simulink library "BLDC_controller_Lib"  (R2017b)
settings: Solver=VariableStepAuto  StartTime=0.0  StopTime=10.0  RelTol=1e-3
undefined symbols (not defined in the file): a_elecAngle, a_elecPeriod, a_phaAdv_M1, b_phaAdvEna, cf_speedCoef, cf_speedFilt, CTRL_COMM, dz_counterHi, dz_counterLo, n_commAcvLo, n_commDeacvHi, n_motPhaAdvEna, r_commDCDeacv, r_sin3PhaA_M1, r_sin3PhaB_M1, r_sin3PhaC_M1, r_sinPhaA_M1, r_sinPhaB_M1, r_sinPhaC_M1, r_trapPhaA_M1, r_trapPhaB_M1, r_trapPhaC_M1, vec_hallToPos, z_commutMap_M1, z_ctrlTypSel, z_maxCntRst
libraries: BLDC_controller_Lib x2, simulink x1
settings Model: Creator=37ef  LastModifiedBy=eferu

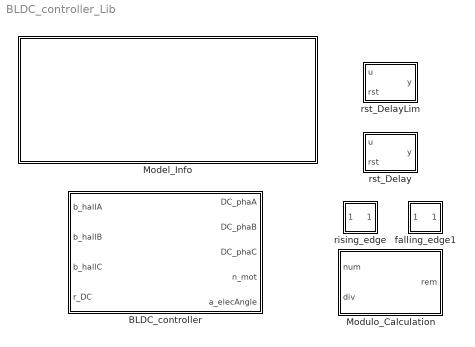
== system BLDC_controller_Lib ==
  BLDC_controller : Subsystem  SystemSampleTime=1e-5
  Model_Info : Subsystem
      mask DialogControl DescGroupVar Prompt: Model info
      mask DialogControl DescTextVar Prompt: This mask gives quick information about the model.
      mask Display:
      | info = Simulink.MDLInfo(bdroot);
      | file = dir([bdroot '.slx']);
      | % image('logo.png', [0.48, 0.55, 0.5, 0.4]);
      | text(0.05, 0.5, [...
      |         'MODEL INFO \n\n' ...
      |         'Version: ' info.ModelVersion '\n' ...
      |         'Author: ' 'Emanuel Feru' '\n' ...
      |         'Last modified by: ' info.LastModifiedBy '\n' ...
      |         'Last update: ' file.date '\n\n'], ...
      |         'horizontalAlignment', 'left', ...
      |         'verticalAlignment', 'middle');
      | 
      | color('blue');
      | text(0.95, 0.08, [...
      |         'Copyright © 2019 Emanuel FERU'], ...
      |         'horizontalAlignment', 'right', ...
      |         'verticalAlignment', 'bottom');
  Modulo_Calculation : Subsystem
  falling_edge1 : Subsystem  StopFcn=%tagged  TreatAsAtomicUnit=on  mask(Falling edge detection){}
      mask help:
      | Falling edge detection for a logic signal.
      | When a falling edge on the input signal is detected, the output switches to 1 during one time step.
      settings: RTWSystemCode=Nonreusable function
      mask Display: plot(0,0,100,100, [20 50 50 80], [90 90 10 10], [40 50 60], [55 45 55] )
  rising_edge : Subsystem  StopFcn=%tagged  TreatAsAtomicUnit=on  mask(Rising edge detection){}
      mask help:
      | Rising edge detection for a logic signal.
      | When a rising edge on the input signal is detected, the output switches to 1 during one time step.
      settings: RTWSystemCode=Nonreusable function
      mask Display: plot(0,0,100,100, [20 50 50 80], [10 10 90 90], [40 50 60], [45 55 45] )
  rst_Delay : Subsystem
      mask Display: dpoly(1,[1 0],'z')
  rst_DelayLim : Subsystem  mask{z_cntMaxLim=200}
      mask prompts: z_cntMaxLim "Maximum counter limit"
      mask Display: dpoly(1,[1 0],'z')

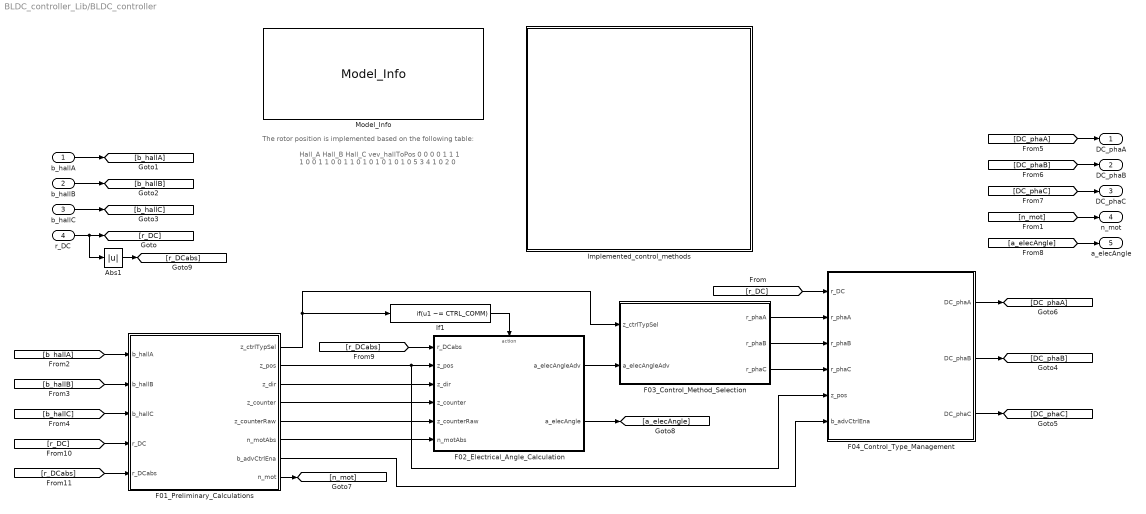
== system BLDC_controller_Lib/BLDC_controller ==
  note: Hall_A
      | Hall_B
      | Hall_C
      | vev_hallToPos
      |
      | 0
      | 0
      | 0
      | 0
      | 1
      | 1
      | 1
      | 1
      | 0
      | 0
      | 1
      | 1
      | 0
      | 0
      | 1
      | 1
      | 0
      | 1
      | 0
      | 1
      | 0
      | 1
      | 0
      | 1
      | 0
      | 5
      | 3
      | 4
      | 1
      | 0
      | 2
      | 0
  note: The rotor position is implemented based on the following table:
  "b_hallA " : Inport
  b_hallB : Inport  Port=2
  b_hallC : Inport  Port=3
  r_DC : Inport  Port=4
  Abs1 : Abs  OutDataTypeStr=Inherit: Inherit via back propagation  RndMeth=Zero
  F01_Preliminary_Calculations : Subsystem
  F02_Electrical_Angle_Calculation : Subsystem
  F03_Control_Method_Selection : Subsystem
  F04_Control_Type_Management : Subsystem
  If1 : If  IfExpression=u1 ~= CTRL_COMM  ShowElse=off
  Implemented_control_methods : Subsystem
      mask Display: image('control_methods.png')
  Model_Info : BLDC_controller_Lib/Model_Info
  DC_phaA : Outport
  DC_phaB : Outport  Port=2
  DC_phaC : Outport  Port=3
  n_mot : Outport  Port=4
  a_elecAngle : Outport  Port=5
  wires:
  F01_Preliminary_Calculations/6(n_motAbs) -> F02_Electrical_Angle_Calculation/6(n_motAbs)
  [r_DCabs] -> F01_Preliminary_Calculations/5(r_DCabs)
  Abs1/1 -> [r_DCabs]
  F01_Preliminary_Calculations/5(z_counterRaw) -> F02_Electrical_Angle_Calculation/5(z_counterRaw)
  F01_Preliminary_Calculations/4(z_counter) -> F02_Electrical_Angle_Calculation/4(z_counter)
  F01_Preliminary_Calculations/7(b_advCtrlEna) -> F04_Control_Type_Management/6(b_advCtrlEna)
  [r_DC] -> F01_Preliminary_Calculations/4(r_DC)
  [r_DCabs] -> F02_Electrical_Angle_Calculation/1(r_DCabs)
  F02_Electrical_Angle_Calculation/2(a_elecAngle) -> [a_elecAngle]
  [a_elecAngle] -> a_elecAngle/1
  r_DC/1 -> Abs1/1, [r_DC]
  [DC_phaC] -> DC_phaC/1
  [DC_phaB] -> DC_phaB/1
  F04_Control_Type_Management/3("DC_phaC ") -> [DC_phaC]
  F04_Control_Type_Management/2(DC_phaB) -> [DC_phaB]
  F04_Control_Type_Management/1(DC_phaA) -> [DC_phaA]
  [r_DC] -> F04_Control_Type_Management/1(r_DC)
  F03_Control_Method_Selection/3("r_phaC ") -> F04_Control_Type_Management/4(r_phaC)
  F03_Control_Method_Selection/2(r_phaB) -> F04_Control_Type_Management/3(r_phaB)
  F03_Control_Method_Selection/1(r_phaA) -> F04_Control_Type_Management/2(r_phaA)
  F02_Electrical_Angle_Calculation/1(a_elecAngleAdv) -> F03_Control_Method_Selection/2(a_elecAngleAdv)
  If1/1 -> F02_Electrical_Angle_Calculation/Action
  F01_Preliminary_Calculations/1(z_ctrlTypSel) -> If1/1, F03_Control_Method_Selection/1(z_ctrlTypSel)
  F01_Preliminary_Calculations/8("n_mot ") -> [n_mot]
  F01_Preliminary_Calculations/3(z_dir) -> F02_Electrical_Angle_Calculation/3(z_dir)
  F01_Preliminary_Calculations/2(z_pos) -> F02_Electrical_Angle_Calculation/2(z_pos), F04_Control_Type_Management/5(z_pos)
  [b_hallB] -> F01_Preliminary_Calculations/2(b_hallB)
  [b_hallC] -> F01_Preliminary_Calculations/3(b_hallC)
  [b_hallA] -> F01_Preliminary_Calculations/1(b_hallA)
  [DC_phaA] -> DC_phaA/1
  [n_mot] -> n_mot/1
  b_hallC/1 -> [b_hallC]
  b_hallB/1 -> [b_hallB]
  "b_hallA "/1 -> [b_hallA]

== system BLDC_controller_Lib/Model_Info ==

== system BLDC_controller_Lib/Modulo_Calculation ==
  note: Modulo implementation: rem = num - div*(num/div)
      | Note : Division and multiplier has the setting 'Floor'
  num : Inport
  div : Inport  Port=2
  Divide2 : Product  Inputs=*/  OutDataTypeStr=Inherit: Same as first input
  Divide3 : Product  Inputs=**  OutDataTypeStr=Inherit: Same as first input
  Sum3 : Sum  Inputs=|+-  RndMeth=Simplest  OutDataTypeStr=Inherit: Same as first input
  rem : Outport
  wires:
  num/1 -> Sum3/1, Divide2/1
  Sum3/1 -> rem/1
  Divide3/1 -> Sum3/2
  div/1 -> Divide3/2, Divide2/2
  Divide2/1 -> Divide3/1

== system BLDC_controller_Lib/falling_edge1 ==
  Signal : Inport
  Logical Operator : Logic  Tag=struct('inputs','2','comment',struct('text','','placement',1),'logdata',struct('maxnumvals',inf,'plotchannels',[],'loggingmode',3,'channels',1),'operator','AND','output',struct('variable','','description','','name','$S_$B','address','','class','default','type','Bool','unit',''),'scalingvalid',0,'date',733067.68453166669)  OutDataTypeStr=boolean
  Logical Operator1 : Logic  Tag=struct('inputs','1','comment',struct('text','','placement',1),'logdata',struct('maxnumvals',inf,'plotchannels',[],'loggingmode',3,'channels',1),'operator','NOT','output',struct('variable','','description','','name','$S_$B','address','','class','default','type','Bool','unit',''),'scalingvalid',0,'date',733067.68453201384)  Operator=NOT  Inputs=1  OutDataTypeStr=boolean
  UnitDelay : UnitDelay  SampleTime=-1
      settings: AttributesFormatString=Te = %<SampleTime>\nIni=%<X0>
  Out : Outport
  wires:
  UnitDelay/1 -> Logical Operator/2
  Logical Operator1/1 -> Logical Operator/1
  Signal/1 -> UnitDelay/1, Logical Operator1/1
  Logical Operator/1 -> Out/1

== system BLDC_controller_Lib/rising_edge ==
  Signal : Inport
  Logical Operator : Logic  Tag=struct('inputs','2','comment',struct('text','','placement',1),'logdata',struct('maxnumvals',inf,'plotchannels',[],'loggingmode',3,'channels',1),'operator','AND','output',struct('variable','','description','','name','$S_$B','address','','class','default','type','Bool','unit',''),'scalingvalid',0,'date',733067.68458487268)  OutDataTypeStr=boolean
  Logical Operator1 : Logic  Tag=struct('inputs','1','comment',struct('text','','placement',1),'logdata',struct('maxnumvals',inf,'plotchannels',[],'loggingmode',3,'channels',1),'operator','NOT','output',struct('variable','','description','','name','$S_$B','address','','class','default','type','Bool','unit',''),'scalingvalid',0,'date',733067.68458533566)  Operator=NOT  Inputs=1  OutDataTypeStr=boolean
  UnitDelay : UnitDelay  SampleTime=-1
      settings: AttributesFormatString=Te = %<SampleTime>\nIni=%<X0>
  Out : Outport
  wires:
  UnitDelay/1 -> Logical Operator1/1
  Logical Operator1/1 -> Logical Operator/2
  Signal/1 -> Logical Operator/1, UnitDelay/1
  Logical Operator/1 -> Out/1

== system BLDC_controller_Lib/rst_Delay ==
  u : Inport
  rst : Inport  Port=2
  Constant23 : Constant  Value=0  OutDataTypeStr=Inherit: Inherit via back propagation
  Switch1 : Switch  Criteria=u2 ~= 0  OutDataTypeStr=Inherit: Inherit via back propagation  RndMeth=Simplest
  UnitDelay1 : UnitDelay  SampleTime=-1
  y : Outport
  wires:
  Switch1/1 -> y/1
  u/1 -> UnitDelay1/1
  UnitDelay1/1 -> Switch1/3
  rst/1 -> Switch1/2
  Constant23/1 -> Switch1/1

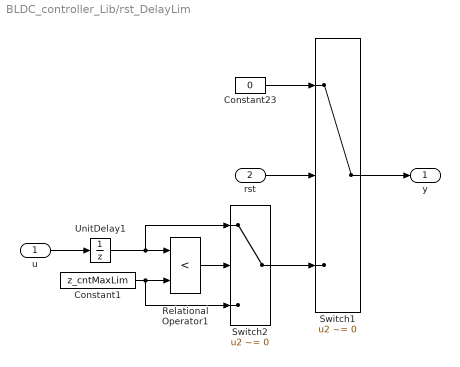
== system BLDC_controller_Lib/rst_DelayLim ==
  u : Inport
  rst : Inport  Port=2
  Constant1 : Constant  Value=z_cntMaxLim  OutDataTypeStr=Inherit: Inherit via back propagation
  Constant23 : Constant  Value=0  OutDataTypeStr=Inherit: Inherit via back propagation
  Relational Operator1 : RelationalOperator  Operator=<  OutDataTypeStr=boolean  RndMeth=Simplest
  Switch1 : Switch  Criteria=u2 ~= 0  OutDataTypeStr=Inherit: Inherit via back propagation  RndMeth=Simplest
  Switch2 : Switch  Criteria=u2 ~= 0  OutDataTypeStr=Inherit: Inherit via back propagation  RndMeth=Simplest
  UnitDelay1 : UnitDelay  InitialCondition=z_cntMaxLim  SampleTime=-1
  y : Outport
  wires:
  Switch1/1 -> y/1
  u/1 -> UnitDelay1/1
  rst/1 -> Switch1/2
  Constant23/1 -> Switch1/1
  UnitDelay1/1 -> Switch2/1, Relational Operator1/1
  Constant1/1 -> Switch2/3, Relational Operator1/2
  Relational Operator1/1 -> Switch2/2
  Switch2/1 -> Switch1/3

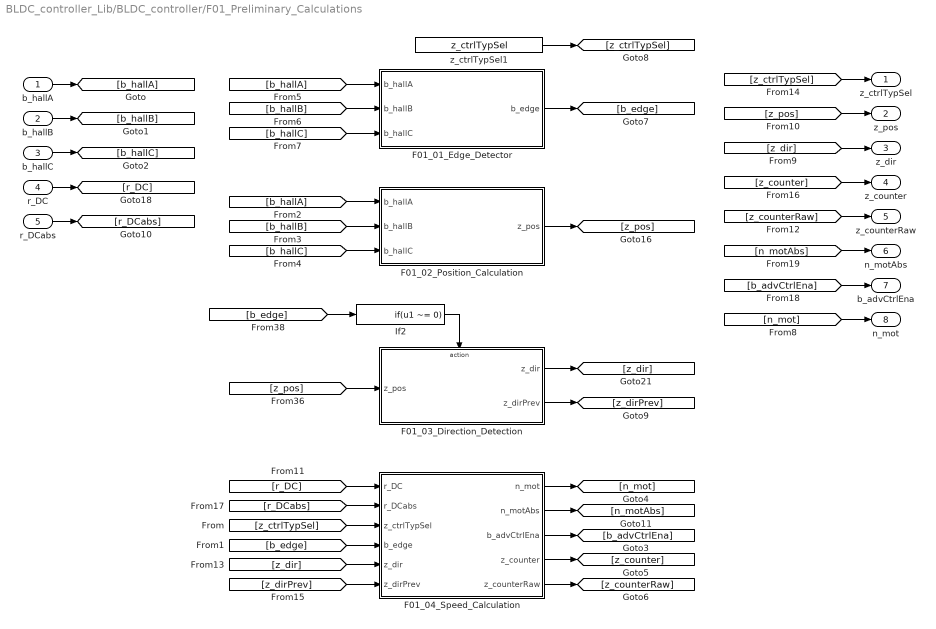
== system BLDC_controller_Lib/BLDC_controller/F01_Preliminary_Calculations ==
  b_hallA : Inport
  b_hallB : Inport  Port=2
  b_hallC : Inport  Port=3
  r_DC : Inport  Port=4
  r_DCabs : Inport  Port=5
  F01_01_Edge_Detector : Subsystem
  F01_02_Position_Calculation : Subsystem
  F01_03_Direction_Detection : Subsystem
  F01_04_Speed_Calculation : Subsystem
  If2 : If  IfExpression=u1 ~= 0  ShowElse=off
  z_ctrlTypSel1 : Constant  Value=z_ctrlTypSel  OutDataTypeStr=uint8
  z_ctrlTypSel : Outport  OutputWhenDisabled=reset  InitialOutput=0
  z_pos : Outport  Port=2  OutputWhenDisabled=reset  InitialOutput=0
  z_dir : Outport  Port=3  OutputWhenDisabled=reset  InitialOutput=0
  z_counter : Outport  Port=4  OutputWhenDisabled=reset  InitialOutput=0
  z_counterRaw : Outport  Port=5  OutputWhenDisabled=reset  InitialOutput=0
  n_motAbs : Outport  Port=6  OutputWhenDisabled=reset  InitialOutput=0
  b_advCtrlEna : Outport  Port=7
  "n_mot " : Outport  Port=8  OutputWhenDisabled=reset  InitialOutput=0
  wires:
  [n_motAbs] -> n_motAbs/1
  F01_04_Speed_Calculation/2(n_motAbs) -> [n_motAbs]
  [r_DCabs] -> F01_04_Speed_Calculation/2(r_DCabs)
  r_DCabs/1 -> [r_DCabs]
  [z_dirPrev] -> F01_04_Speed_Calculation/6(z_dirPrev)
  F01_03_Direction_Detection/2(z_dirPrev) -> [z_dirPrev]
  F01_04_Speed_Calculation/5(z_counterRaw) -> [z_counterRaw]
  F01_04_Speed_Calculation/4(z_counter) -> [z_counter]
  [z_counterRaw] -> z_counterRaw/1
  [z_counter] -> z_counter/1
  F01_04_Speed_Calculation/3(b_advCtrlEna) -> [b_advCtrlEna]
  [b_advCtrlEna] -> b_advCtrlEna/1
  [r_DC] -> F01_04_Speed_Calculation/1(r_DC)
  [z_ctrlTypSel] -> F01_04_Speed_Calculation/3(z_ctrlTypSel)
  r_DC/1 -> [r_DC]
  z_ctrlTypSel1/1 -> [z_ctrlTypSel]
  [z_ctrlTypSel] -> z_ctrlTypSel/1
  [z_dir] -> F01_04_Speed_Calculation/5(z_dir)
  [z_pos] -> z_pos/1
  [z_dir] -> z_dir/1
  [n_mot] -> "n_mot "/1
  F01_04_Speed_Calculation/1(n_mot) -> [n_mot]
  [b_edge] -> F01_04_Speed_Calculation/4(b_edge)
  F01_02_Position_Calculation/1("z_pos ") -> [z_pos]
  [b_hallA] -> F01_02_Position_Calculation/1(b_hallA)
  [b_hallB] -> F01_02_Position_Calculation/2(b_hallB)
  [b_hallC] -> F01_02_Position_Calculation/3(b_hallC)
  b_hallC/1 -> [b_hallC]
  b_hallB/1 -> [b_hallB]
  b_hallA/1 -> [b_hallA]
  [b_hallC] -> F01_01_Edge_Detector/3(b_hallC)
  [b_hallB] -> F01_01_Edge_Detector/2(b_hallB)
  F01_03_Direction_Detection/1(z_dir) -> [z_dir]
  F01_01_Edge_Detector/1("b_edge ") -> [b_edge]
  [b_hallA] -> F01_01_Edge_Detector/1(b_hallA)
  [z_pos] -> F01_03_Direction_Detection/1(z_pos)
  [b_edge] -> If2/1
  If2/1 -> F01_03_Direction_Detection/Action

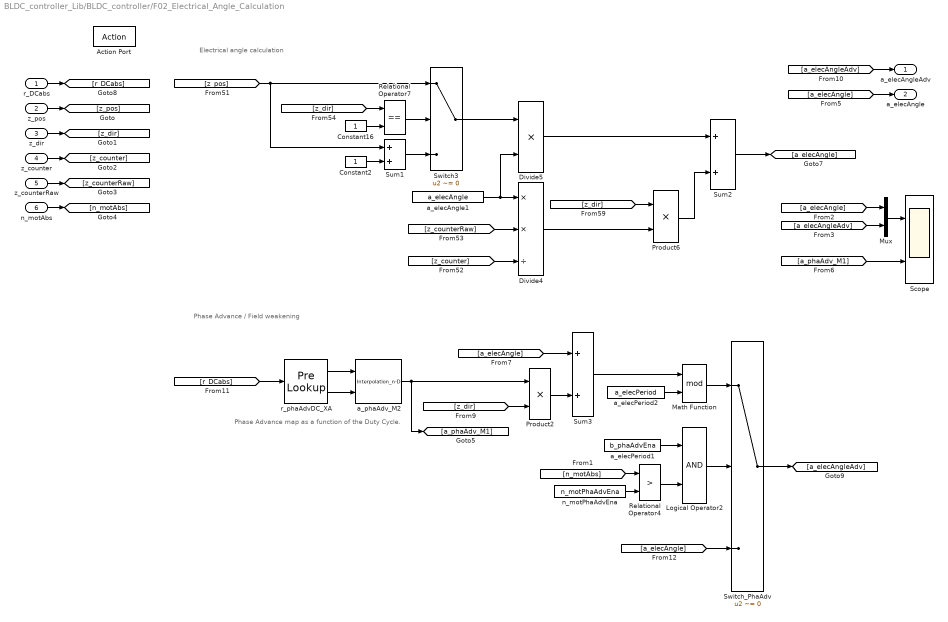
== system BLDC_controller_Lib/BLDC_controller/F02_Electrical_Angle_Calculation ==
  note: Phase Advance map as a function of the Duty Cycle.
  note: Phase Advance / Field weakening
  note: Electrical angle calculation
  r_DCabs : Inport
  z_pos : Inport  Port=2
  z_dir : Inport  Port=3
  z_counter : Inport  Port=4
  z_counterRaw : Inport  Port=5
  n_motAbs : Inport  Port=6
  Action Port : ActionPort
  Constant16 : Constant  OutDataTypeStr=Inherit: Inherit via back propagation
  Constant2 : Constant  OutDataTypeStr=Inherit: Inherit via back propagation
  Divide4 : Product  Inputs=**/  OutDataTypeStr=int32  RndMeth=Simplest
  Divide5 : Product  Inputs=**  OutDataTypeStr=int32  RndMeth=Simplest
  Logical Operator2 : Logic  AllPortsSameDT=off  OutDataTypeStr=boolean
  Math Function : Math  Operator=mod  SaturateOnIntegerOverflow=on
  Mux : Mux  Inputs=2
  Product2 : Product  RndMeth=Simplest  OutDataTypeStr=Inherit: Same as first input
  Product6 : Product  OutDataTypeStr=Inherit: Inherit via back propagation  RndMeth=Simplest
  Relational Operator4 : RelationalOperator  Operator=>  OutDataTypeStr=boolean  RndMeth=Simplest
  Relational Operator7 : RelationalOperator  Operator===  OutDataTypeStr=boolean  RndMeth=Simplest
  Scope : Scope  NumInputPorts=2
  Sum1 : Sum  RndMeth=Simplest  OutDataTypeStr=Inherit: Same as first input
  Sum2 : Sum  RndMeth=Simplest  OutDataTypeStr=Inherit: Same as first input
  Sum3 : Sum  RndMeth=Simplest  OutDataTypeStr=Inherit: Same as first input
  Switch3 : Switch  Criteria=u2 ~= 0  OutDataTypeStr=Inherit: Inherit via back propagation  RndMeth=Zero
  Switch_PhaAdv : Switch  Criteria=u2 ~= 0  OutDataTypeStr=Inherit: Inherit via back propagation  RndMeth=Zero
  a_elecAngle1 : Constant  Value=a_elecAngle  OutDataTypeStr=int32
  a_elecPeriod1 : Constant  Value=b_phaAdvEna  OutDataTypeStr=boolean
  a_elecPeriod2 : Constant  Value=a_elecPeriod  OutDataTypeStr=Inherit: Inherit via back propagation
  a_phaAdv_M2 : Interpolation_n-D  NumberOfTableDimensions=1  Table=a_phaAdv_M1  ExtrapMethod=Clip  OutDataTypeStr=int16  InternalRulePriority=Speed  RndMeth=Simplest
      settings: InputPortMap=u0,u1
  n_motPhaAdvEna : Constant  Value=n_motPhaAdvEna  OutDataTypeStr=Inherit: Inherit via back propagation
  r_phaAdvDC_XA : PreLookup  BreakpointsData=r_phaAdvDC_XA  IndexSearchMethod=Evenly spaced points  BeginIndexSearchUsingPreviousIndexResult=on  IndexDataTypeStr=uint8  RndMeth=Simplest
  a_elecAngleAdv : Outport  OutputWhenDisabled=reset  InitialOutput=0
  a_elecAngle : Outport  Port=2  OutputWhenDisabled=reset  InitialOutput=0
  wires:
  n_motAbs/1 -> [n_motAbs]
  Logical Operator2/1 -> Switch_PhaAdv/2
  Relational Operator4/1 -> Logical Operator2/2
  [n_motAbs] -> Relational Operator4/1
  n_motPhaAdvEna/1 -> Relational Operator4/2
  a_elecPeriod1/1 -> Logical Operator2/1
  Divide5/1 -> Sum2/1
  Divide4/1 -> Product6/2
  Sum1/1 -> Switch3/3
  [z_dir] -> Relational Operator7/1
  a_elecAngle1/1 -> Divide4/1, Divide5/2
  Constant16/1 -> Relational Operator7/2
  Relational Operator7/1 -> Switch3/2
  Product6/1 -> Sum2/2
  [z_counter] -> Divide4/3
  Constant2/1 -> Sum1/2
  [z_pos] -> Sum1/1, Switch3/1
  Sum2/1 -> [a_elecAngle]
  [z_dir] -> Product6/1
  Switch3/1 -> Divide5/1
  [z_counterRaw] -> Divide4/2
  z_counter/1 -> [z_counter]
  z_counterRaw/1 -> [z_counterRaw]
  Sum3/1 -> Math Function/1
  Math Function/1 -> Switch_PhaAdv/1
  a_elecPeriod2/1 -> Math Function/2
  [r_DCabs] -> r_phaAdvDC_XA/1
  [a_elecAngle] -> Sum3/1
  Product2/1 -> Sum3/2
  Switch_PhaAdv/1 -> [a_elecAngleAdv]
  r_DCabs/1 -> [r_DCabs]
  [a_elecAngle] -> Switch_PhaAdv/3
  r_phaAdvDC_XA/1 -> a_phaAdv_M2/1
  r_phaAdvDC_XA/2 -> a_phaAdv_M2/2
  [a_phaAdv_M1] -> Scope/2
  [a_elecAngleAdv] -> a_elecAngleAdv/1
  [a_elecAngle] -> a_elecAngle/1
  [a_elecAngleAdv] -> Mux/2
  [a_elecAngle] -> Mux/1
  Mux/1 -> Scope/1
  z_dir/1 -> [z_dir]
  z_pos/1 -> [z_pos]
  [z_dir] -> Product2/2
  a_phaAdv_M2/1 -> Product2/1, [a_phaAdv_M1]

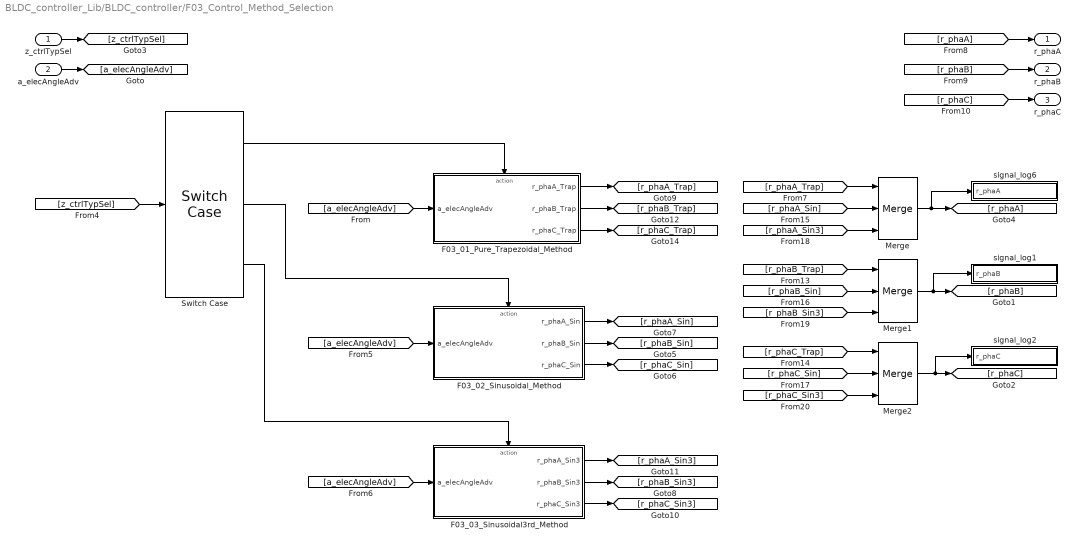
== system BLDC_controller_Lib/BLDC_controller/F03_Control_Method_Selection ==
  z_ctrlTypSel : Inport
  a_elecAngleAdv : Inport  Port=2
  F03_01_Pure_Trapezoidal_Method : Subsystem
  F03_02_Sinusoidal_Method : Subsystem
  F03_03_Sinusoidal3rd_Method : Subsystem
  Merge : Merge  Inputs=3
  Merge1 : Merge  Inputs=3
  Merge2 : Merge  Inputs=3
  Switch Case : SwitchCase  CaseConditions={CTRL_TRAP, CTRL_SIN, CTRL_SIN3}  ShowDefaultCase=off
  signal_log1 : Subsystem
  signal_log2 : Subsystem
  signal_log6 : Subsystem
  r_phaA : Outport  OutputWhenDisabled=reset  InitialOutput=0
  r_phaB : Outport  Port=2  OutputWhenDisabled=reset  InitialOutput=0
  "r_phaC " : Outport  Port=3  OutputWhenDisabled=reset  InitialOutput=0
  wires:
  [r_phaC_Sin3] -> Merge2/3
  [r_phaC_Sin] -> Merge2/2
  [r_phaB_Sin3] -> Merge1/3
  [r_phaC_Trap] -> Merge2/1
  [r_phaB_Sin] -> Merge1/2
  [r_phaB_Trap] -> Merge1/1
  [r_phaA_Sin3] -> Merge/3
  [r_phaA_Sin] -> Merge/2
  z_ctrlTypSel/1 -> [z_ctrlTypSel]
  [r_phaA_Trap] -> Merge/1
  Merge2/1 -> [r_phaC], signal_log2/1(r_phaC)
  Merge1/1 -> [r_phaB], signal_log1/1(r_phaB)
  Merge/1 -> [r_phaA], signal_log6/1(r_phaA)
  F03_03_Sinusoidal3rd_Method/1(r_phaA_Sin3) -> [r_phaA_Sin3]
  F03_03_Sinusoidal3rd_Method/2(r_phaB_Sin3) -> [r_phaB_Sin3]
  F03_03_Sinusoidal3rd_Method/3(r_phaC_Sin3) -> [r_phaC_Sin3]
  F03_02_Sinusoidal_Method/1(r_phaA_Sin) -> [r_phaA_Sin]
  F03_02_Sinusoidal_Method/2(r_phaB_Sin) -> [r_phaB_Sin]
  F03_02_Sinusoidal_Method/3(r_phaC_Sin) -> [r_phaC_Sin]
  F03_01_Pure_Trapezoidal_Method/3(r_phaC_Trap) -> [r_phaC_Trap]
  F03_01_Pure_Trapezoidal_Method/2(r_phaB_Trap) -> [r_phaB_Trap]
  Switch Case/3 -> F03_03_Sinusoidal3rd_Method/Action
  Switch Case/2 -> F03_02_Sinusoidal_Method/Action
  [a_elecAngleAdv] -> F03_03_Sinusoidal3rd_Method/1(a_elecAngleAdv)
  [a_elecAngleAdv] -> F03_02_Sinusoidal_Method/1(a_elecAngleAdv)
  Switch Case/1 -> F03_01_Pure_Trapezoidal_Method/Action
  [a_elecAngleAdv] -> F03_01_Pure_Trapezoidal_Method/1(a_elecAngleAdv)
  [z_ctrlTypSel] -> Switch Case/1
  F03_01_Pure_Trapezoidal_Method/1(r_phaA_Trap) -> [r_phaA_Trap]
  a_elecAngleAdv/1 -> [a_elecAngleAdv]
  [r_phaC] -> "r_phaC "/1
  [r_phaB] -> r_phaB/1
  [r_phaA] -> r_phaA/1

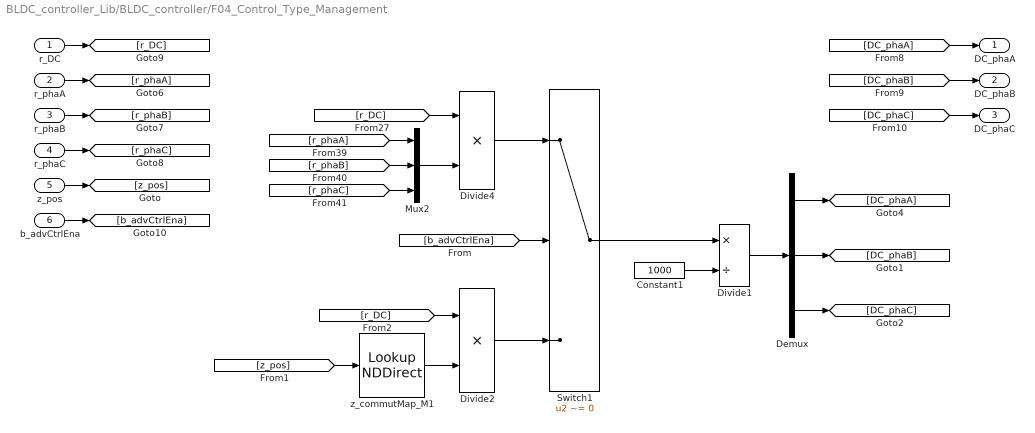
== system BLDC_controller_Lib/BLDC_controller/F04_Control_Type_Management ==
  r_DC : Inport
  r_phaA : Inport  Port=2
  r_phaB : Inport  Port=3
  r_phaC : Inport  Port=4
  z_pos : Inport  Port=5
  b_advCtrlEna : Inport  Port=6
  Constant1 : Constant  Value=1000  OutDataTypeStr=Inherit: Inherit via back propagation
  Demux : Demux  Outputs=3
  Divide1 : Product  Inputs=*/  RndMeth=Simplest  OutDataTypeStr=Inherit: Same as first input
  Divide2 : Product  Inputs=**  RndMeth=Simplest  OutDataTypeStr=Inherit: Same as first input
  Divide4 : Product  Inputs=**  RndMeth=Simplest  OutDataTypeStr=Inherit: Same as first input
  Mux2 : Mux  Inputs=3
  Switch1 : Switch  Criteria=u2 ~= 0  OutDataTypeStr=Inherit: Inherit via back propagation  RndMeth=Zero
  z_commutMap_M1 : LookupNDDirect  InputsSelectThisObjectFromTable=Column  Table=z_commutMap_M1  DiagnosticForOutOfRangeInput=None  TableDataTypeStr=int16
  DC_phaA : Outport  OutputWhenDisabled=reset  InitialOutput=0
  DC_phaB : Outport  Port=2  OutputWhenDisabled=reset  InitialOutput=0
  "DC_phaC " : Outport  Port=3  OutputWhenDisabled=reset  InitialOutput=0
  wires:
  [b_advCtrlEna] -> Switch1/2
  b_advCtrlEna/1 -> [b_advCtrlEna]
  [r_DC] -> Divide4/1
  Divide2/1 -> Switch1/3
  z_commutMap_M1/1 -> Divide2/2
  [r_DC] -> Divide2/1
  Constant1/1 -> Divide1/2
  Divide4/1 -> Switch1/1
  Mux2/1 -> Divide4/2
  [r_phaC] -> Mux2/3
  [r_phaB] -> Mux2/2
  [r_phaA] -> Mux2/1
  r_DC/1 -> [r_DC]
  r_phaC/1 -> [r_phaC]
  r_phaB/1 -> [r_phaB]
  r_phaA/1 -> [r_phaA]
  Divide1/1 -> Demux/1
  [z_pos] -> z_commutMap_M1/1
  Switch1/1 -> Divide1/1
  [DC_phaA] -> DC_phaA/1
  [DC_phaB] -> DC_phaB/1
  [DC_phaC] -> "DC_phaC "/1
  z_pos/1 -> [z_pos]
  Demux/1 -> [DC_phaA]
  Demux/2 -> [DC_phaB]
  Demux/3 -> [DC_phaC]

== system BLDC_controller_Lib/BLDC_controller/Implemented_control_methods ==

== system BLDC_controller_Lib/BLDC_controller/F01_Preliminary_Calculations/F01_01_Edge_Detector ==
  b_hallA : Inport
  b_hallB : Inport  Port=2
  b_hallC : Inport  Port=3
  Bitwise Operator : simulink/Logic and Bit Operations/Bitwise Operator  logicop=XOR  UseBitMask=off  NumInputPorts=6  BitMask=bin2dec('11011001')  BitMaskRealWorld=Stored Integer
  UnitDelay : UnitDelay  SampleTime=-1
  UnitDelay1 : UnitDelay  SampleTime=-1
  UnitDelay2 : UnitDelay  SampleTime=-1
  "b_edge " : Outport  OutputWhenDisabled=reset  InitialOutput=0
  wires:
  UnitDelay/1 -> Bitwise Operator/4
  UnitDelay2/1 -> Bitwise Operator/6
  UnitDelay1/1 -> Bitwise Operator/5
  Bitwise Operator/1 -> "b_edge "/1
  b_hallB/1 -> UnitDelay1/1, Bitwise Operator/2
  b_hallC/1 -> UnitDelay2/1, Bitwise Operator/3
  b_hallA/1 -> UnitDelay/1, Bitwise Operator/1

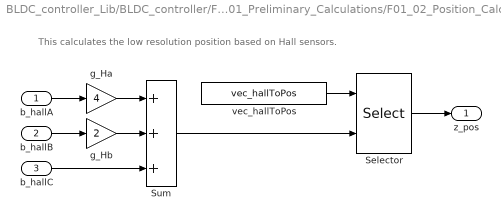
== system BLDC_controller_Lib/BLDC_controller/F01_Preliminary_Calculations/F01_02_Position_Calculation ==
  note: This calculates the low resolution position based on Hall sensors.
  b_hallA : Inport
  b_hallB : Inport  Port=2
  b_hallC : Inport  Port=3
  Selector : Selector  IndexMode=Zero-based  InputPortWidth=length(vec_hallToPos)  IndexOptions=Index vector (port)  Indices=[1 3]  OutputSizes=1
  Sum : Sum  Inputs=+++  RndMeth=Simplest  OutDataTypeStr=Inherit: Same as first input
  g_Ha : Gain  Gain=4  OutDataTypeStr=Inherit: Inherit via back propagation  RndMeth=Zero  ParamDataTypeStr=Inherit: Same as input
  g_Hb : Gain  Gain=2  OutDataTypeStr=Inherit: Inherit via back propagation  RndMeth=Simplest  ParamDataTypeStr=Inherit: Same as input
  vec_hallToPos : Constant  Value=vec_hallToPos  OutDataTypeStr=int8
  "z_pos " : Outport  OutputWhenDisabled=reset  InitialOutput=0
  wires:
  Selector/1 -> "z_pos "/1
  vec_hallToPos/1 -> Selector/1
  b_hallB/1 -> g_Hb/1
  b_hallA/1 -> g_Ha/1
  Sum/1 -> Selector/2
  g_Hb/1 -> Sum/2
  g_Ha/1 -> Sum/1
  b_hallC/1 -> Sum/3

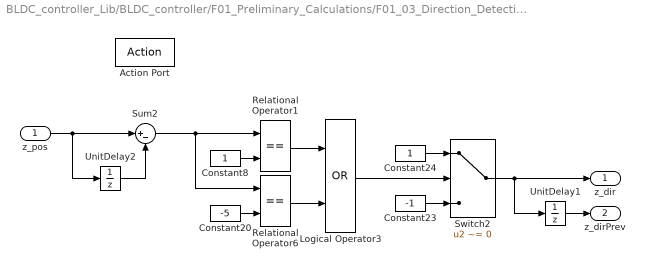
== system BLDC_controller_Lib/BLDC_controller/F01_Preliminary_Calculations/F01_03_Direction_Detection ==
  z_pos : Inport
  Action Port : ActionPort
  Constant20 : Constant  Value=-5  OutDataTypeStr=Inherit: Inherit via back propagation
  Constant23 : Constant  Value=-1  OutDataTypeStr=int8
  Constant24 : Constant  OutDataTypeStr=int8
  Constant8 : Constant  OutDataTypeStr=Inherit: Inherit via back propagation
  Logical Operator3 : Logic  Operator=OR  AllPortsSameDT=off  OutDataTypeStr=boolean
  Relational Operator1 : RelationalOperator  Operator===  OutDataTypeStr=boolean  RndMeth=Simplest
  Relational Operator6 : RelationalOperator  Operator===  OutDataTypeStr=boolean  RndMeth=Simplest
  Sum2 : Sum  Inputs=|+-  RndMeth=Zero  InputSameDT=on  OutDataTypeStr=Inherit: Same as first input
  Switch2 : Switch  Criteria=u2 ~= 0  OutDataTypeStr=Inherit: Inherit via back propagation  RndMeth=Simplest
  UnitDelay1 : UnitDelay  SampleTime=-1
  UnitDelay2 : UnitDelay  SampleTime=-1
  z_dir : Outport
  z_dirPrev : Outport  Port=2
  wires:
  UnitDelay1/1 -> z_dirPrev/1
  Switch2/1 -> z_dir/1, UnitDelay1/1
  z_pos/1 -> UnitDelay2/1, Sum2/1
  Logical Operator3/1 -> Switch2/2
  Constant23/1 -> Switch2/3
  Constant24/1 -> Switch2/1
  Constant20/1 -> Relational Operator6/2
  Relational Operator6/1 -> Logical Operator3/2
  Sum2/1 -> Relational Operator1/1, Relational Operator6/1
  Constant8/1 -> Relational Operator1/2
  Relational Operator1/1 -> Logical Operator3/1
  UnitDelay2/1 -> Sum2/2

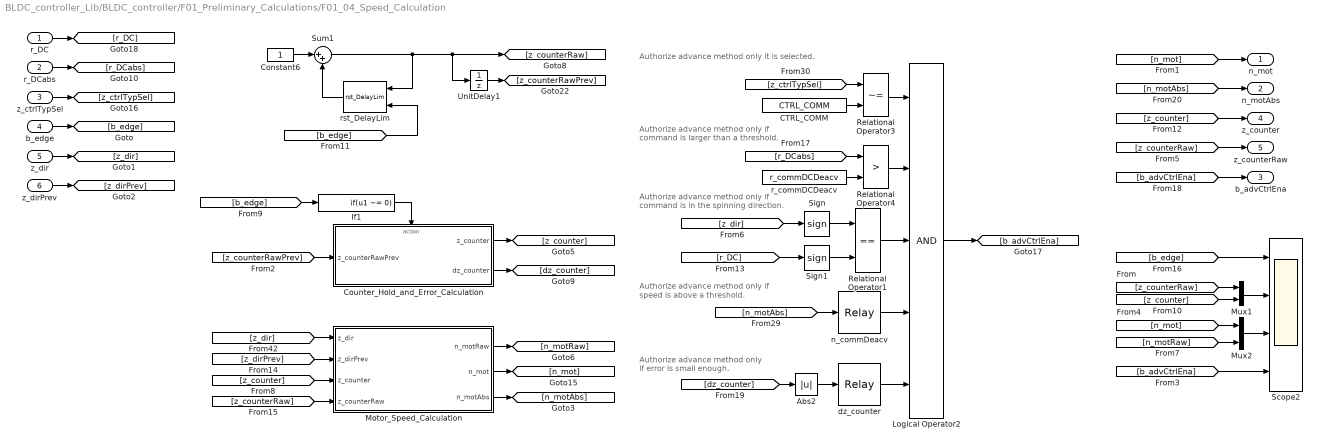
== system BLDC_controller_Lib/BLDC_controller/F01_Preliminary_Calculations/F01_04_Speed_Calculation ==
  note: Authorize advance method only it is selected.
  note: Authorize advance method only if command is larger than a threshold.
  note: Authorize advance method only if error is small enough.
  note: Authorize advance method only if command is in the spinning direction.
  note: Authorize advance method only if speed is above a threshold.
  r_DC : Inport
  r_DCabs : Inport  Port=2
  z_ctrlTypSel : Inport  Port=3
  b_edge : Inport  Port=4
  z_dir : Inport  Port=5
  z_dirPrev : Inport  Port=6
  Abs2 : Abs  OutDataTypeStr=Inherit: Inherit via back propagation  RndMeth=Zero
  CTRL_COMM : Constant  Value=CTRL_COMM  OutDataTypeStr=Inherit: Inherit via back propagation
  Constant6 : Constant  OutDataTypeStr=int16
  Counter_Hold_and_Error_Calculation : Subsystem
  If1 : If  IfExpression=u1 ~= 0  ShowElse=off
  Logical Operator2 : Logic  Inputs=5  AllPortsSameDT=off  OutDataTypeStr=boolean
  Motor_Speed_Calculation : Subsystem
  Mux1 : Mux  Inputs=2
  Mux2 : Mux  Inputs=2
  Relational Operator1 : RelationalOperator  Operator===  OutDataTypeStr=boolean  RndMeth=Simplest
  Relational Operator3 : RelationalOperator  Operator=~=  OutDataTypeStr=boolean  RndMeth=Simplest
  Relational Operator4 : RelationalOperator  Operator=>  OutDataTypeStr=boolean  RndMeth=Simplest
  Scope2 : Scope  NumInputPorts=4
  Sign : Signum
  Sign1 : Signum
  Sum1 : Sum  Inputs=|++  RndMeth=Simplest  InputSameDT=on  OutDataTypeStr=Inherit: Same as first input
  UnitDelay1 : UnitDelay  SampleTime=-1
  dz_counter : Relay  OnSwitchValue=dz_counterHi  OffSwitchValue=dz_counterLo  OnOutputValue=0  OffOutputValue=1  OutDataTypeStr=boolean
  n_commDeacv : Relay  OnSwitchValue=n_commDeacvHi  OffSwitchValue=n_commAcvLo  OutDataTypeStr=boolean
  r_commDCDeacv : Constant  Value=r_commDCDeacv  OutDataTypeStr=Inherit: Inherit via back propagation
  rst_DelayLim : BLDC_controller_Lib/rst_DelayLim  z_cntMaxLim=z_maxCntRst
  n_mot : Outport
  n_motAbs : Outport  Port=2
  b_advCtrlEna : Outport  Port=3
  z_counter : Outport  Port=4  OutputWhenDisabled=reset  InitialOutput=0
  z_counterRaw : Outport  Port=5  OutputWhenDisabled=reset  InitialOutput=0
  wires:
  [n_motAbs] -> n_motAbs/1
  Motor_Speed_Calculation/3(n_motAbs) -> [n_motAbs]
  r_DCabs/1 -> [r_DCabs]
  Relational Operator1/1 -> Logical Operator2/3
  Relational Operator4/1 -> Logical Operator2/2
  Relational Operator3/1 -> Logical Operator2/1
  n_commDeacv/1 -> Logical Operator2/4
  [z_counterRaw] -> Motor_Speed_Calculation/4(z_counterRaw)
  [z_dirPrev] -> Motor_Speed_Calculation/2(z_dirPrev)
  z_dirPrev/1 -> [z_dirPrev]
  [b_edge] -> If1/1
  Sign1/1 -> Relational Operator1/2
  [r_DC] -> Sign1/1
  Sign/1 -> Relational Operator1/1
  [z_dir] -> Sign/1
  [b_advCtrlEna] -> Scope2/4
  UnitDelay1/1 -> [z_counterRawPrev]
  [b_edge] -> rst_DelayLim/2
  [z_counterRaw] -> z_counterRaw/1
  [z_counter] -> z_counter/1
  [z_counter] -> Motor_Speed_Calculation/3(z_counter)
  Motor_Speed_Calculation/1(n_motRaw) -> [n_motRaw]
  Motor_Speed_Calculation/2(n_mot) -> [n_mot]
  [z_dir] -> Motor_Speed_Calculation/1(z_dir)
  [b_advCtrlEna] -> b_advCtrlEna/1
  r_DC/1 -> [r_DC]
  z_ctrlTypSel/1 -> [z_ctrlTypSel]
  [dz_counter] -> Abs2/1
  Counter_Hold_and_Error_Calculation/2(dz_counter) -> [dz_counter]
  [z_counterRawPrev] -> Counter_Hold_and_Error_Calculation/1(z_counterRawPrev)
  Counter_Hold_and_Error_Calculation/1(z_counter) -> [z_counter]
  If1/1 -> Counter_Hold_and_Error_Calculation/Action
  Logical Operator2/1 -> [b_advCtrlEna]
  r_commDCDeacv/1 -> Relational Operator4/2
  [r_DCabs] -> Relational Operator4/1
  CTRL_COMM/1 -> Relational Operator3/2
  [n_motAbs] -> n_commDeacv/1
  [z_ctrlTypSel] -> Relational Operator3/1
  rst_DelayLim/1 -> Sum1/2
  z_dir/1 -> [z_dir]
  [n_mot] -> n_mot/1
  b_edge/1 -> [b_edge]
  Sum1/1 -> UnitDelay1/1, [z_counterRaw], rst_DelayLim/1
  Constant6/1 -> Sum1/1
  [b_edge] -> Scope2/1
  [z_counter] -> Mux1/2
  [z_counterRaw] -> Mux1/1
  Mux1/1 -> Scope2/2
  [n_mot] -> Mux2/1
  Mux2/1 -> Scope2/3
  [n_motRaw] -> Mux2/2
  dz_counter/1 -> Logical Operator2/5
  Abs2/1 -> dz_counter/1

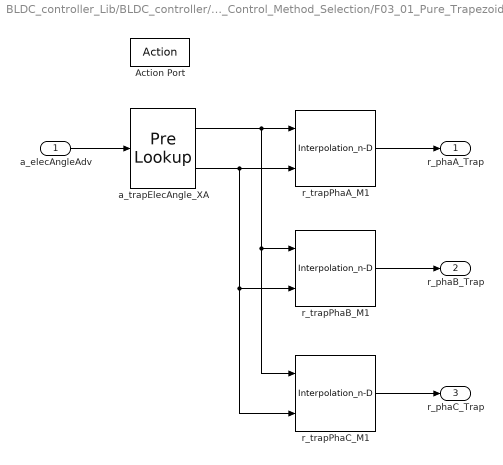
== system BLDC_controller_Lib/BLDC_controller/F03_Control_Method_Selection/F03_01_Pure_Trapezoidal_Method ==
  a_elecAngleAdv : Inport
  Action Port : ActionPort  InitializeStates=reset
  a_trapElecAngle_XA : PreLookup  BreakpointsData=a_trapElecAngle_XA  IndexSearchMethod=Evenly spaced points  BeginIndexSearchUsingPreviousIndexResult=on  IndexDataTypeStr=uint8  RndMeth=Simplest
  r_trapPhaA_M1 : Interpolation_n-D  NumberOfTableDimensions=1  Table=r_trapPhaA_M1  ExtrapMethod=Clip  RemoveProtectionIndex=on  OutDataTypeStr=int16  InternalRulePriority=Speed  RndMeth=Simplest
      settings: InputPortMap=u0,u1
  r_trapPhaB_M1 : Interpolation_n-D  NumberOfTableDimensions=1  Table=r_trapPhaB_M1  ExtrapMethod=Clip  RemoveProtectionIndex=on  OutDataTypeStr=int16  InternalRulePriority=Speed  RndMeth=Simplest
      settings: InputPortMap=u0,u1
  r_trapPhaC_M1 : Interpolation_n-D  NumberOfTableDimensions=1  Table=r_trapPhaC_M1  ExtrapMethod=Clip  RemoveProtectionIndex=on  OutDataTypeStr=int16  InternalRulePriority=Speed  RndMeth=Simplest
      settings: InputPortMap=u0,u1
  r_phaA_Trap : Outport
  r_phaB_Trap : Outport  Port=2
  r_phaC_Trap : Outport  Port=3
  wires:
  a_elecAngleAdv/1 -> a_trapElecAngle_XA/1
  r_trapPhaC_M1/1 -> r_phaC_Trap/1
  r_trapPhaB_M1/1 -> r_phaB_Trap/1
  r_trapPhaA_M1/1 -> r_phaA_Trap/1
  a_trapElecAngle_XA/2 -> r_trapPhaA_M1/2, r_trapPhaB_M1/2, r_trapPhaC_M1/2
  a_trapElecAngle_XA/1 -> r_trapPhaB_M1/1, r_trapPhaC_M1/1, r_trapPhaA_M1/1

== system BLDC_controller_Lib/BLDC_controller/F03_Control_Method_Selection/F03_02_Sinusoidal_Method ==
  a_elecAngleAdv : Inport
  Action Port : ActionPort  InitializeStates=reset
  a_sinElecAngle_XA : PreLookup  BreakpointsData=a_sinElecAngle_XA  IndexSearchMethod=Evenly spaced points  BeginIndexSearchUsingPreviousIndexResult=on  IndexDataTypeStr=uint8  RndMeth=Simplest
  r_sinPhaA_M1 : Interpolation_n-D  NumberOfTableDimensions=1  Table=r_sinPhaA_M1  ExtrapMethod=Clip  RemoveProtectionIndex=on  OutDataTypeStr=int16  InternalRulePriority=Speed  RndMeth=Simplest
      settings: InputPortMap=u0,u1
  r_sinPhaB_M1 : Interpolation_n-D  NumberOfTableDimensions=1  Table=r_sinPhaB_M1  ExtrapMethod=Clip  RemoveProtectionIndex=on  OutDataTypeStr=int16  InternalRulePriority=Speed  RndMeth=Simplest
      settings: InputPortMap=u0,u1
  r_sinPhaC_M1 : Interpolation_n-D  NumberOfTableDimensions=1  Table=r_sinPhaC_M1  ExtrapMethod=Clip  RemoveProtectionIndex=on  OutDataTypeStr=int16  InternalRulePriority=Speed  RndMeth=Simplest
      settings: InputPortMap=u0,u1
  r_phaA_Sin : Outport
  r_phaB_Sin : Outport  Port=2
  r_phaC_Sin : Outport  Port=3
  wires:
  a_sinElecAngle_XA/1 -> r_sinPhaC_M1/1, r_sinPhaB_M1/1, r_sinPhaA_M1/1
  r_sinPhaA_M1/1 -> r_phaA_Sin/1
  r_sinPhaB_M1/1 -> r_phaB_Sin/1
  r_sinPhaC_M1/1 -> r_phaC_Sin/1
  a_elecAngleAdv/1 -> a_sinElecAngle_XA/1
  a_sinElecAngle_XA/2 -> r_sinPhaC_M1/2, r_sinPhaB_M1/2, r_sinPhaA_M1/2

== system BLDC_controller_Lib/BLDC_controller/F03_Control_Method_Selection/F03_03_Sinusoidal3rd_Method ==
  a_elecAngleAdv : Inport
  Action Port : ActionPort  InitializeStates=reset
  a_sinElecAngle_XA : PreLookup  BreakpointsData=a_sinElecAngle_XA  IndexSearchMethod=Evenly spaced points  BeginIndexSearchUsingPreviousIndexResult=on  IndexDataTypeStr=uint8  RndMeth=Simplest
  r_sin3PhaA_M1 : Interpolation_n-D  NumberOfTableDimensions=1  Table=r_sin3PhaA_M1  ExtrapMethod=Clip  RemoveProtectionIndex=on  OutDataTypeStr=int16  InternalRulePriority=Speed  RndMeth=Simplest
      settings: InputPortMap=u0,u1
  r_sin3PhaB_M1 : Interpolation_n-D  NumberOfTableDimensions=1  Table=r_sin3PhaB_M1  ExtrapMethod=Clip  RemoveProtectionIndex=on  OutDataTypeStr=int16  InternalRulePriority=Speed  RndMeth=Simplest
      settings: InputPortMap=u0,u1
  r_sin3PhaC_M1 : Interpolation_n-D  NumberOfTableDimensions=1  Table=r_sin3PhaC_M1  ExtrapMethod=Clip  RemoveProtectionIndex=on  OutDataTypeStr=int16  InternalRulePriority=Speed  RndMeth=Simplest
      settings: InputPortMap=u0,u1
  r_phaA_Sin3 : Outport
  r_phaB_Sin3 : Outport  Port=2
  r_phaC_Sin3 : Outport  Port=3
  wires:
  a_elecAngleAdv/1 -> a_sinElecAngle_XA/1
  r_sin3PhaC_M1/1 -> r_phaC_Sin3/1
  r_sin3PhaB_M1/1 -> r_phaB_Sin3/1
  r_sin3PhaA_M1/1 -> r_phaA_Sin3/1
  a_sinElecAngle_XA/2 -> r_sin3PhaA_M1/2, r_sin3PhaB_M1/2, r_sin3PhaC_M1/2
  a_sinElecAngle_XA/1 -> r_sin3PhaB_M1/1, r_sin3PhaC_M1/1, r_sin3PhaA_M1/1

== system BLDC_controller_Lib/BLDC_controller/F03_Control_Method_Selection/signal_log1 ==
  r_phaB : Inport
  Terminator_1 : Terminator
  wires:
  r_phaB/1 -> Terminator_1/1  "r_phaB"

== system BLDC_controller_Lib/BLDC_controller/F03_Control_Method_Selection/signal_log2 ==
  r_phaC : Inport
  Terminator_1 : Terminator
  wires:
  r_phaC/1 -> Terminator_1/1  "r_phaC"

== system BLDC_controller_Lib/BLDC_controller/F03_Control_Method_Selection/signal_log6 ==
  r_phaA : Inport
  Terminator_1 : Terminator
  wires:
  r_phaA/1 -> Terminator_1/1  "r_phaA"

== system BLDC_controller_Lib/BLDC_controller/F01_Preliminary_Calculations/F01_04_Speed_Calculation/Counter_Hold_and_Error_Calculation ==
  z_counterRawPrev : Inport
  Action Port : ActionPort
  Sum4 : Sum  Inputs=+-  RndMeth=Simplest  InputSameDT=on  OutDataTypeStr=Inherit: Same as first input
  z_counter2 : UnitDelay  InitialCondition=z_maxCntRst  SampleTime=-1
  z_counter : Outport  InitialOutput=z_maxCntRst
  dz_counter : Outport  Port=2
  wires:
  Sum4/1 -> dz_counter/1
  z_counter2/1 -> Sum4/2
  z_counterRawPrev/1 -> z_counter/1, Sum4/1, z_counter2/1

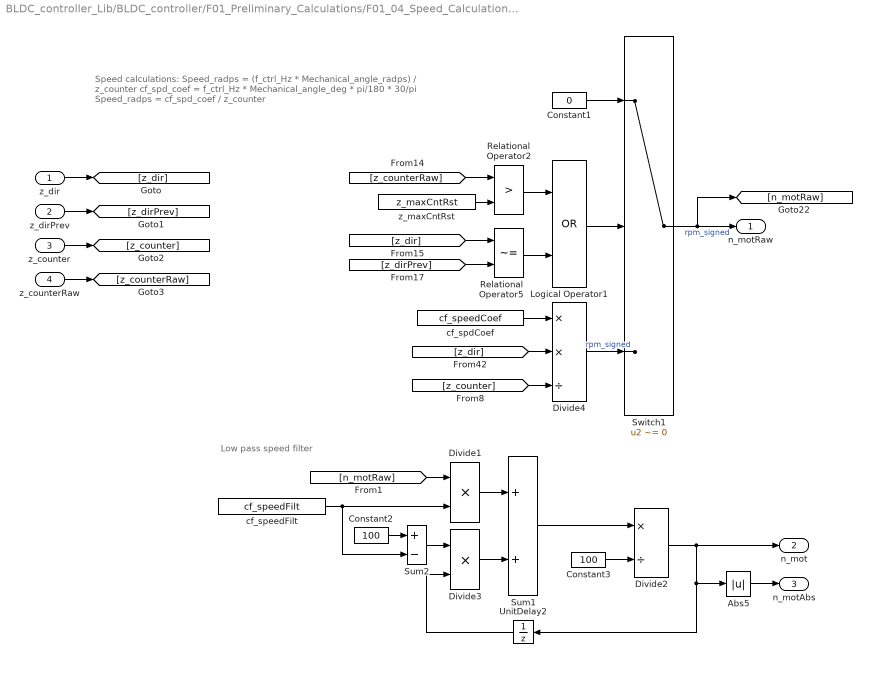
== system BLDC_controller_Lib/BLDC_controller/F01_Preliminary_Calculations/F01_04_Speed_Calculation/Motor_Speed_Calculation ==
  note: Speed calculations:
      | Speed_radps = (f_ctrl_Hz * Mechanical_angle_radps) / z_counter
      | cf_spd_coef = f_ctrl_Hz * Mechanical_angle_deg * pi/180 * 30/pi
      | Speed_radps = cf_spd_coef / z_counter
  note: Low pass speed filter
  z_dir : Inport
  z_dirPrev : Inport  Port=2
  z_counter : Inport  Port=3
  z_counterRaw : Inport  Port=4
  Abs5 : Abs  OutDataTypeStr=Inherit: Inherit via back propagation  RndMeth=Zero
  Constant1 : Constant  Value=0  OutDataTypeStr=Inherit: Inherit via back propagation
  Constant2 : Constant  Value=100  OutDataTypeStr=Inherit: Inherit via back propagation
  Constant3 : Constant  Value=100  OutDataTypeStr=Inherit: Inherit via back propagation
  Divide1 : Product  Inputs=**  RndMeth=Simplest  OutDataTypeStr=Inherit: Same as first input
  Divide2 : Product  Inputs=*/  RndMeth=Simplest  OutDataTypeStr=Inherit: Same as first input
  Divide3 : Product  Inputs=**  RndMeth=Simplest  OutDataTypeStr=Inherit: Same as first input
  Divide4 : Product  Inputs=**/  RndMeth=Simplest  OutDataTypeStr=Inherit: Same as first input
  Logical Operator1 : Logic  Operator=OR  AllPortsSameDT=off  OutDataTypeStr=boolean
  Relational Operator2 : RelationalOperator  Operator=>  OutDataTypeStr=boolean  RndMeth=Simplest
  Relational Operator5 : RelationalOperator  Operator=~=  OutDataTypeStr=boolean  RndMeth=Simplest
  Sum1 : Sum  RndMeth=Simplest  InputSameDT=on  OutDataTypeStr=Inherit: Same as first input
  Sum2 : Sum  Inputs=+-  RndMeth=Simplest  InputSameDT=on  OutDataTypeStr=Inherit: Same as first input
  Switch1 : Switch  Criteria=u2 ~= 0  OutDataTypeStr=Inherit: Inherit via back propagation  RndMeth=Zero
  UnitDelay2 : UnitDelay  SampleTime=-1
  cf_spdCoef : Constant  Value=cf_speedCoef  OutDataTypeStr=int32
  cf_speedFilt : Constant  Value=cf_speedFilt  OutDataTypeStr=int32
  z_maxCntRst : Constant  Value=z_maxCntRst  OutDataTypeStr=Inherit: Inherit via back propagation
  n_motRaw : Outport
  n_mot : Outport  Port=2
  n_motAbs : Outport  Port=3
  wires:
  Abs5/1 -> n_motAbs/1
  z_counterRaw/1 -> [z_counterRaw]
  z_counter/1 -> [z_counter]
  z_dirPrev/1 -> [z_dirPrev]
  z_dir/1 -> [z_dir]
  Divide4/1 -> Switch1/3  "rpm_signed"
  Constant1/1 -> Switch1/1
  Logical Operator1/1 -> Switch1/2
  Relational Operator5/1 -> Logical Operator1/2
  [z_counterRaw] -> Relational Operator2/1
  [z_dirPrev] -> Relational Operator5/2
  [z_dir] -> Relational Operator5/1
  z_maxCntRst/1 -> Relational Operator2/2
  Relational Operator2/1 -> Logical Operator1/1
  [z_dir] -> Divide4/2
  Constant3/1 -> Divide2/2
  Sum1/1 -> Divide2/1
  Divide2/1 -> Abs5/1, UnitDelay2/1, n_mot/1
  Divide1/1 -> Sum1/1
  UnitDelay2/1 -> Divide3/2
  [z_counter] -> Divide4/3
  cf_spdCoef/1 -> Divide4/1
  Switch1/1 -> [n_motRaw], n_motRaw/1  "rpm_signed"
  Divide3/1 -> Sum1/2
  Constant2/1 -> Sum2/1
  Sum2/1 -> Divide3/1
  cf_speedFilt/1 -> Sum2/2, Divide1/2
  [n_motRaw] -> Divide1/1
